simulink library "FUSA_EM_EMRL"  (R2023b)
settings: Solver=VariableStepAuto  StartTime=0.0  StopTime=10.0  RelTol=1e-3
undefined symbols (not defined in the file): FUSA_EM_EMRL_p1_TempMotDertCoefReLe_na, FUSA_EM_EMRL_px_TempMotReLeLkp_degC
libraries: simulink x1
settings Model: Creator=blatak  LastModifiedBy=blatak

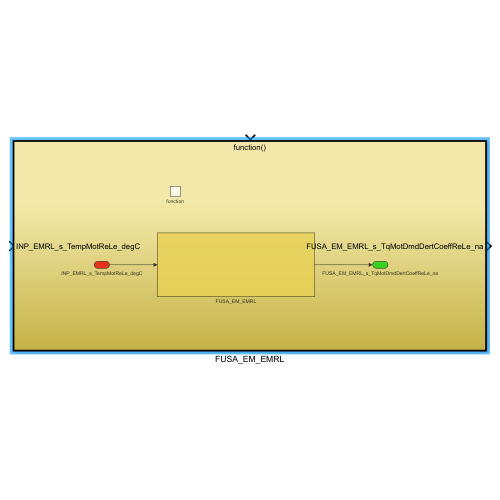
[thumbnail: Simulink's stored preview of the top-level diagram]
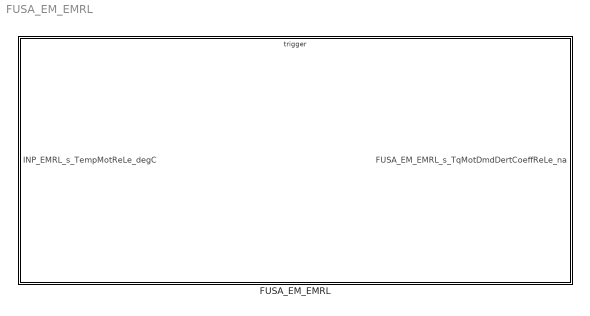
== system FUSA_EM_EMRL ==
  FUSA_EM_EMRL : Subsystem  TreatAsAtomicUnit=on

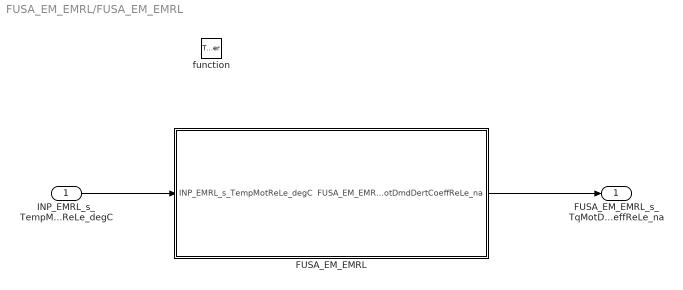
== system FUSA_EM_EMRL/FUSA_EM_EMRL ==
  INP_EMRL_s_TempMotReLe_degC : Inport
  function : TriggerPort  TriggerType=function-call  VariantControl=(inherit)
  FUSA_EM_EMRL : Subsystem
  FUSA_EM_EMRL_s_TqMotDmdDertCoeffReLe_na : Outport  Description=Derate torque coefficient front
  wires:
  INP_EMRL_s_TempMotReLe_degC/1 -> FUSA_EM_EMRL/1(INP_EMRL_s_TempMotReLe_degC)
  FUSA_EM_EMRL/1(FUSA_EM_EMRL_s_TqMotDmdDertCoeffReLe_na) -> FUSA_EM_EMRL_s_TqMotDmdDertCoeffReLe_na/1

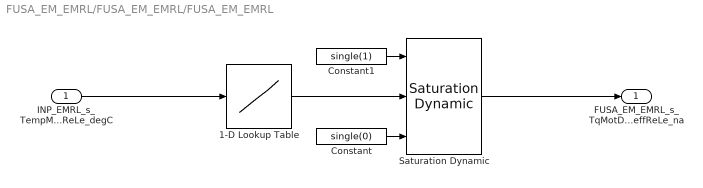
== system FUSA_EM_EMRL/FUSA_EM_EMRL/FUSA_EM_EMRL ==
  INP_EMRL_s_TempMotReLe_degC : Inport
  1-D Lookup Table : Lookup_n-D  NumberOfTableDimensions=1  BreakpointsForDimension1=FUSA_EM_EMRL_px_TempMotReLeLkp_degC  Table=FUSA_EM_EMRL_p1_TempMotDertCoefReLe_na  InternalRulePriority=Speed  RndMeth=Simplest
  Constant : Constant  Value=single(0)
  Constant1 : Constant  Value=single(1)
  Saturation Dynamic : simulink/Discontinuities/Saturation Dynamic  OutMin=[]  OutMax=[]  OutDataTypeStr=Inherit: Same as second input  OutDataType=fixdt(1, 16)  OutScaling=2^-10  DoSatur=off
  FUSA_EM_EMRL_s_TqMotDmdDertCoeffReLe_na : Outport  Description=Derate torque coefficient front
  wires:
  Constant/1 -> Saturation Dynamic/3
  Constant1/1 -> Saturation Dynamic/1
  1-D Lookup Table/1 -> Saturation Dynamic/2
  Saturation Dynamic/1 -> FUSA_EM_EMRL_s_TqMotDmdDertCoeffReLe_na/1
  INP_EMRL_s_TempMotReLe_degC/1 -> 1-D Lookup Table/1
